simulink model "PMSM_speedcontrol"  (R2023a)
settings: Solver=VariableStepAuto  StartTime=0.0  StopTime=0.5  RelTol=1e-3
libraries: spsMosfetLib x6, simulink x3, spsDCVoltageSourceLib x1, spsPermanentMagnetSynchronousMachineLib x1, spsSawtoothGeneratorLib x1, spsThreePhaseVIMeasurementLib x1, sps_lib x1, spspowerguiLib x1
settings Model: Creator=Ganesh Fashion  LastModifiedBy=Ganesh Fashion

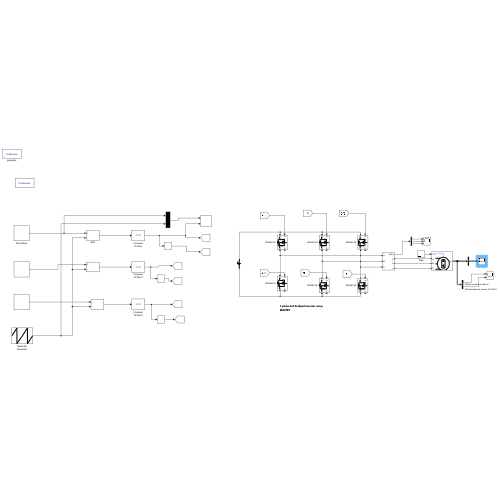
[thumbnail: Simulink's stored preview of the top-level diagram]
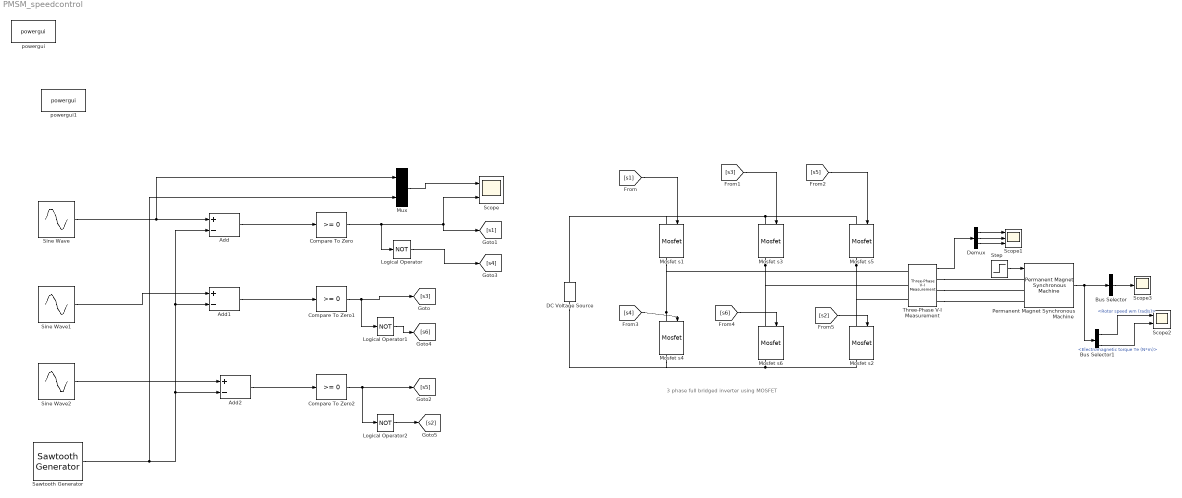
== system PMSM_speedcontrol ==
  note: 3 phase full bridged inverter using MOSFET
  Add : Sum  Inputs=+-
  Add1 : Sum  Inputs=+-
  Add2 : Sum  Inputs=+-
  Bus Selector : BusSelector  OutputSignals=Stator current is_a (A),Stator current is_c (A),Stator current is_b (A)  OutputAsBus=on
  Bus Selector1 : BusSelector  OutputSignals=Rotor speed wm (rad/s),Electromagnetic torque Te (N*m)
  Compare To Zero : simulink/Logic and Bit Operations/Compare To Zero  relop=>=  OutDataTypeStr=boolean
  Compare To Zero1 : simulink/Logic and Bit Operations/Compare To Zero  relop=>=  OutDataTypeStr=boolean
  Compare To Zero2 : simulink/Logic and Bit Operations/Compare To Zero  relop=>=  OutDataTypeStr=boolean
  DC Voltage Source : spsDCVoltageSourceLib/DC Voltage Source  Amplitude=300  Measurements=None
  Demux : Demux  Outputs=3
  Logical Operator : Logic  Operator=NOT  AllPortsSameDT=off  OutDataTypeStr=boolean
  Logical Operator1 : Logic  Operator=NOT  AllPortsSameDT=off  OutDataTypeStr=boolean
  Logical Operator2 : Logic  Operator=NOT  AllPortsSameDT=off  OutDataTypeStr=boolean
  Mosfet s{1..6} (6 alike) : spsMosfetLib/Mosfet  Ron=0.1  Lon=0  Rd=0.01  Vfd=0  IC=0  Rs=1e5  Cs=inf  Measurements=on
  Mux : Mux  Inputs=2
  Permanent Magnet Synchronous Machine : spsPermanentMagnetSynchronousMachineLib/Permanent Magnet Synchronous Machine  NbPhases=3  FluxDistribution=Sinusoidal  RotorType=Round  MechanicalLoad=Torque Tm  PresetModel=No  ShowDetailedParameters=on  MeasurementBus=off  Resistance=4.765  Inductance=8.5e-3  dqInductances=[8.5e-3,8.5e-3]  La=0.014  MachineConstant=Flux linkage established by magnets (V.s)  Flux=0.1848  VoltageCst=67.038  TorqueCst=0.5544  Flat=120  Mechanical=[0.0001051 4.047e-05 2 0]  PolePairs=2  InitialConditions=[0,0, 0,0]  InitialConditions5ph=[0 0 0 0 0 0]  RefAngle=90 degrees behind phase A axis (modified Park)  IterativeDiscreteModel=Trapezoidal non iterative  TsBlock=-1  TsPowergui=0
  Sawtooth Generator : spsSawtoothGeneratorLib/Sawtooth Generator  Freq=1e3  Phase=180  Ts=0
  Scope : Scope  NumInputPorts=2
  Scope1 : Scope  NumInputPorts=3
  Scope2 : Scope  NumInputPorts=2
  Scope3 : Scope
  Sine Wave : Sin  Frequency=2*pi*50  SampleTime=0
  Sine Wave1 : Sin  Frequency=2*pi*50  Phase=2*pi/3  SampleTime=0
  Sine Wave2 : Sin  Frequency=2*pi*50  Phase=4*pi/3  SampleTime=0
  Step : Step  Time=0.2  After=3  SampleTime=0  ZeroCross=off
  Three-Phase V-I Measurement : spsThreePhaseVIMeasurementLib/Three-Phase V-I Measurement  VoltageMeasurement=phase-to-phase  SetLabelV=off  LabelV=Vabc  Vpu=off  VpuLL=off  CurrentMeasurement=no  SetLabelI=off  LabelI=Iabc  Ipu=off  Pbase=100e6  Vbase=500e3  OutputType=Complex  PhasorSimulation=off  PSBequivalent=0
  powergui : sps_lib/powergui  Priority=1  SimulationMode=Continuous  SampleTime=50e-6  frequency=60  Iterations=50  frequencyindice=0  Pbase=100e6  ErrMax=1e-4  UnitsV=kV  UnitsW=MW  buscounter=0  FunctionMessages=off  echomessages=off  EnableUseOfTLC=off  CurrentSourceSwitches=off  DisableSnubberDevices=off  DisableRonSwitches=off  DisableVfSwitches=off  DisplayEquations=off  AutomaticDiscreteSolvers=off  SolverType=Tustin/Backward Euler (TBE)  Interpol=off  ExternalGateDelay=off  methode=off  Ts=100  x0status=blocks  SPID=on  SwTol=0  HookPort=off  NonlinearTolerance=1e-4  nMaxIteration=100  ContinueOnMaxIteration=off  RestoreLinks=warning  ResistiveCurrentMeasurement=off  Frange=[0:2:500]  Ylog=off  Xlog=on  ShowGrid=off  save=off  variable=ZData  structure=0  ZoomFFT=off  StartTime=0.0  cycles=1  DisplayStyle=1  fundamental=60  FreqAxis=off  MaxFrequency=1000  frequencyindicesteady=1  RmsSteady=1  display=off
  powergui1 : spspowerguiLib/powergui  Priority=1  SimulationMode=Continuous  SampleTime=50e-6  frequency=60  Iterations=50  frequencyindice=0  Pbase=100e6  ErrMax=1e-4  UnitsV=kV  UnitsW=MW  buscounter=0  FunctionMessages=off  echomessages=off  EnableUseOfTLC=off  CurrentSourceSwitches=off  DisableSnubberDevices=off  DisableRonSwitches=off  DisableVfSwitches=off  DisplayEquations=off  AutomaticDiscreteSolvers=off  SolverType=Tustin/Backward Euler (TBE)  Interpol=off  ExternalGateDelay=off  methode=off  Ts=100  x0status=blocks  SPID=on  SwTol=0  HookPort=off  NonlinearTolerance=1e-4  nMaxIteration=100  ContinueOnMaxIteration=off  RestoreLinks=warning  ResistiveCurrentMeasurement=off  Frange=[0:2:500]  Ylog=off  Xlog=on  ShowGrid=off  save=off  variable=ZData  structure=0  ZoomFFT=off  StartTime=0.0  cycles=1  DisplayStyle=1  fundamental=60  FreqAxis=off  MaxFrequency=1000  frequencyindicesteady=1  RmsSteady=1  display=off
  wires:
  [s5] -> Mosfet s5/1
  [s3] -> Mosfet s3/1
  Logical Operator/1 -> [s4]
  Compare To Zero/1 -> Logical Operator/1, Scope/2, [s1]
  Sine Wave1/1 -> Add1/1
  Sine Wave2/1 -> Add2/1
  Demux/2 -> Scope1/2
  Demux/1 -> Scope1/1
  Three-Phase V-I Measurement/1 -> Demux/1
  Logical Operator1/1 -> [s6]
  [s1] -> Mosfet s1/1
  Mux/1 -> Scope/1
  Add1/1 -> Compare To Zero1/1
  [s6] -> Mosfet s6/1
  Compare To Zero1/1 -> Logical Operator1/1, [s3]
  Add2/1 -> Compare To Zero2/1
  [s4] -> Mosfet s4/1
  Sawtooth Generator/1 -> Add2/2, Add1/2, Add/2, Mux/2
  [s2] -> Mosfet s2/1
  Demux/3 -> Scope1/3
  Sine Wave/1 -> Mux/1, Add/1
  Add/1 -> Compare To Zero/1
  Compare To Zero2/1 -> Logical Operator2/1, [s5]
  Logical Operator2/1 -> [s2]
  Permanent Magnet Synchronous Machine/1 -> Bus Selector/1, Bus Selector1/1
  Bus Selector1/1 -> Scope2/1  "<Rotor speed wm (rad/s)>"
  Bus Selector1/2 -> Scope2/2  "<Electromagnetic torque Te (N*m)>"
  Bus Selector/1 -> Scope3/1
  Step/1 -> Permanent Magnet Synchronous Machine/1
  connections:
  Mosfet s6/RConn1 -- Mosfet s2/RConn1 -- Mosfet s4/RConn1 -- DC Voltage Source/LConn1
  Mosfet s4/LConn1 -- Mosfet s1/RConn1 -- Three-Phase V-I Measurement/LConn1
  Mosfet s5/RConn1 -- Mosfet s2/LConn1 -- Three-Phase V-I Measurement/LConn3
  Mosfet s3/LConn1 -- Mosfet s1/LConn1 -- DC Voltage Source/RConn1 -- Mosfet s5/LConn1
  Mosfet s3/RConn1 -- Mosfet s6/LConn1 -- Three-Phase V-I Measurement/LConn2
  Three-Phase V-I Measurement/RConn2 -- Permanent Magnet Synchronous Machine/LConn2
  Three-Phase V-I Measurement/RConn3 -- Permanent Magnet Synchronous Machine/LConn3
  Three-Phase V-I Measurement/RConn1 -- Permanent Magnet Synchronous Machine/LConn1
